simulink model "PMSM_temperature_estimation_EKF"  (R2023b)
settings: Solver=VariableStepAuto  StartTime=0.0  StopTime=10  FixedStep=dt  RelTol=1e-3  AbsTol=1e-3
values from neighbouring files (symbols this model uses):
  CF_fc = 1/(20*Ts)    (= 5)    [controller_parameters.m]
  CF_k = 1    [controller_parameters.m]
  dt = 50e-6    (= 5e-05)    [config.m]
  dt_speed_control = 0.001    [config.m]
  max_power = 50e3    (= 50000)    [config.m]
  max_torque = 220    [config.m]
  N = 6    [config.m]
  ratio_rotor = 0.75    [config.m]
  Rd_percent_rotor = ratio_rotor*100    (= 75)    [config.m]
  Rm_percent_rotor = ratio_rotor*100    (= 75)    [config.m]
  rotor_initial_temperatures = 298.15    [config.m]
  stator_initial_temperatures = [298.15;298.15;298.15]    [config.m]
  stator_thermal_mass = 100    [config.m]
  Ts = 0.01    [controller_parameters.m]
undefined symbols (not defined in the file or in its folder): cex, ch, cJ, DiscIntNeverNeededParam
libraries: fl_lib x152, nesl_utility x45, fl_ps_legacy_lib x3, sharedTrackingLibrary x1, ee_lib x1, SignalEditorBlockLib x1, simulink x1
(part 2 of 3)

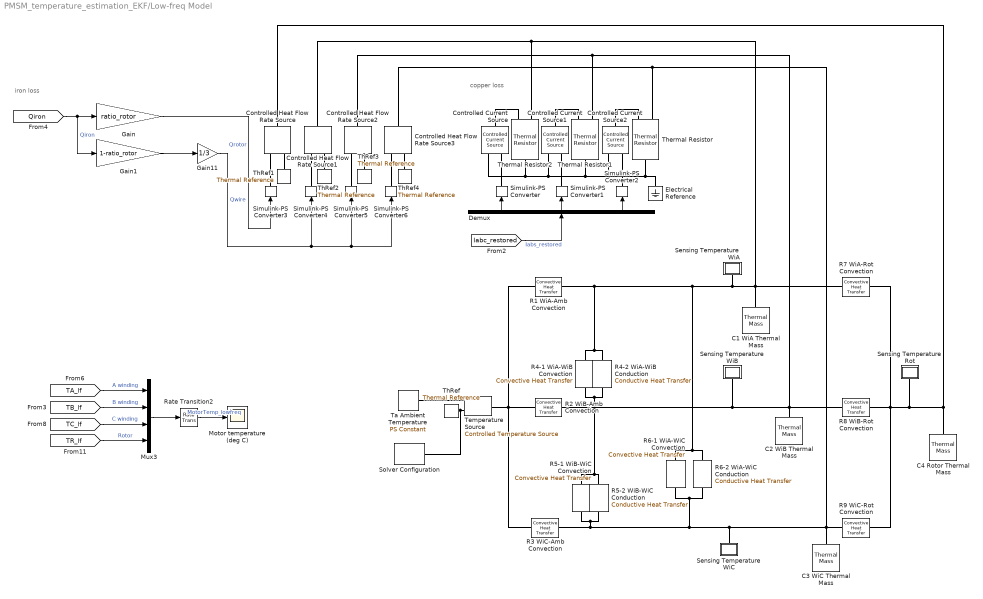
== system PMSM_temperature_estimation_EKF/Low-freq Model ==
  note: iron loss
  note: copper loss
  C1 WiA Thermal Mass : fl_lib/Thermal/Thermal Elements/Thermal Mass  mass_type=foundation.enum.constant_variable.constant  mass=1 kg  sp_heat=stator_thermal_mass J/(K*kg)  mass_min=1e-6 kg  num_ports=foundation.enum.numPorts2.one  m_specify=off  m_priority=High  m=1 kg  m_nominal_specify=off  m_nominal_unit=kg  m_nominal_value=1  T_specify=on  T_priority=High  T=stator_initial_temperatures(1) K  T_nominal_specify=off  T_nominal_unit=K  T_nominal_value=1  Q_specify=off  Q_priority=High  Q=0 W  Q_nominal_specify=off  Q_nominal_unit=W  Q_nominal_value=1
  C2 WiB Thermal Mass : fl_lib/Thermal/Thermal Elements/Thermal Mass  mass_type=foundation.enum.constant_variable.constant  mass=1 kg  sp_heat=stator_thermal_mass J/(K*kg)  mass_min=1e-6 kg  num_ports=foundation.enum.numPorts2.one  m_specify=off  m_priority=High  m=1 kg  m_nominal_specify=off  m_nominal_unit=kg  m_nominal_value=1  T_specify=on  T_priority=High  T=stator_initial_temperatures(2) K  T_nominal_specify=off  T_nominal_unit=K  T_nominal_value=1  Q_specify=off  Q_priority=High  Q=0 W  Q_nominal_specify=off  Q_nominal_unit=W  Q_nominal_value=1
  C3 WiC Thermal Mass : fl_lib/Thermal/Thermal Elements/Thermal Mass  mass_type=foundation.enum.constant_variable.constant  mass=1 kg  sp_heat=stator_thermal_mass J/(K*kg)  mass_min=1e-6 kg  num_ports=foundation.enum.numPorts2.one  m_specify=off  m_priority=High  m=1 kg  m_nominal_specify=off  m_nominal_unit=kg  m_nominal_value=1  T_specify=on  T_priority=High  T=stator_initial_temperatures(3) K  T_nominal_specify=off  T_nominal_unit=K  T_nominal_value=1  Q_specify=off  Q_priority=High  Q=0 W  Q_nominal_specify=off  Q_nominal_unit=W  Q_nominal_value=1
  C4 Rotor Thermal Mass : fl_lib/Thermal/Thermal Elements/Thermal Mass  mass_type=foundation.enum.constant_variable.constant  mass=1 kg  sp_heat=rotor_thermal_mass J/(K*kg)  mass_min=1e-6 kg  num_ports=foundation.enum.numPorts2.one  m_specify=off  m_priority=High  m=1 kg  m_nominal_specify=off  m_nominal_unit=kg  m_nominal_value=1  T_specify=on  T_priority=High  T=rotor_initial_temperatures K  T_nominal_specify=off  T_nominal_unit=K  T_nominal_value=1  Q_specify=off  Q_priority=High  Q=0 W  Q_nominal_specify=off  Q_nominal_unit=W  Q_nominal_value=1
  Controlled Current Source : fl_lib/Electrical/Electrical Sources/Controlled Current Source
  Controlled Current Source1 : fl_lib/Electrical/Electrical Sources/Controlled Current Source
  Controlled Current Source2 : fl_lib/Electrical/Electrical Sources/Controlled Current Source
  Controlled Heat Flow Rate Source{,1..3} (4 alike) : fl_lib/Thermal/Thermal Sources/Controlled Heat Flow Rate Source
  Demux : Demux  Outputs=3
  Electrical Reference : fl_lib/Electrical/Electrical Elements/Electrical Reference
  Gain : Gain  Gain=ratio_rotor
  Gain1 : Gain  Gain=1-ratio_rotor
  Gain11 : Gain  Gain=1/3
  Motor temperature (deg C) : Scope
  Mux3 : Mux
  R1 WiA-Amb Convection : fl_lib/Thermal/Thermal Elements/Convective Heat Transfer  thermal_type=foundation.enum.constant_variable.constant  area=0.1 m^2  heat_tr_coeff=20 W/(m^2 * K)  min_heat_tr_coeff=1e-3 W/(K*m^2)  T_specify=off  T_priority=None  T=0 K  T_nominal_specify=off  T_nominal_unit=K  T_nominal_value=1  Q_specify=off  Q_priority=None  Q=0 J/s  Q_nominal_specify=off  Q_nominal_unit=J/s  Q_nominal_value=1
  R2 WiB-Amb Convection : fl_lib/Thermal/Thermal Elements/Convective Heat Transfer  thermal_type=foundation.enum.constant_variable.constant  area=0.1 m^2  heat_tr_coeff=20 W/(m^2 * K)  min_heat_tr_coeff=1e-3 W/(K*m^2)  T_specify=off  T_priority=None  T=0 K  T_nominal_specify=off  T_nominal_unit=K  T_nominal_value=1  Q_specify=off  Q_priority=None  Q=0 J/s  Q_nominal_specify=off  Q_nominal_unit=J/s  Q_nominal_value=1
  R3 WiC-Amb Convection : fl_lib/Thermal/Thermal Elements/Convective Heat Transfer  thermal_type=foundation.enum.constant_variable.constant  area=0.1 m^2  heat_tr_coeff=20 W/(m^2 * K)  min_heat_tr_coeff=1e-3 W/(K*m^2)  T_specify=off  T_priority=None  T=0 K  T_nominal_specify=off  T_nominal_unit=K  T_nominal_value=1  Q_specify=off  Q_priority=None  Q=0 J/s  Q_nominal_specify=off  Q_nominal_unit=J/s  Q_nominal_value=1
  R4-1 WiA-WiB Convection : fl_lib/Thermal/Thermal Elements/Convective Heat Transfer  thermal_type=foundation.enum.constant_variable.constant  area=0.004 m^2  heat_tr_coeff=200 W/(m^2 * K)  min_heat_tr_coeff=1e-3 W/(K*m^2)  T_specify=off  T_priority=None  T=0 K  T_nominal_specify=off  T_nominal_unit=K  T_nominal_value=1  Q_specify=off  Q_priority=None  Q=0 J/s  Q_nominal_specify=off  Q_nominal_unit=J/s  Q_nominal_value=1
  R4-2 WiA-WiB Conduction : fl_lib/Thermal/Thermal Elements/Conductive Heat Transfer  thermal_type=foundation.enum.ConstantVariableTabulated.Constant  wall_geometry=foundation.enum.ConductionWallGeometry.Planar  area=0.002 m^2  thickness=0.1 m  d_in=0.05 m  d_out=0.1 m  L=1 m  th_cond_min=10 W/(K*m)  th_cond=80 W/(m*K)  th_cond_TLU=[413, 401, 392, 383, 371, 357, 342] W/(K*m)  temp_TLU=[200, 273, 400, 600, 800, 1000, 1200] K  T_specify=off  T_priority=None  T=0 K  T_nominal_specify=off  T_nominal_unit=K  T_nominal_value=1  Q_specify=off  Q_priority=None  Q=0 J/s  Q_nominal_specify=off  Q_nominal_unit=J/s  Q_nominal_value=1
  R5-1 WiB-WiC Convection : fl_lib/Thermal/Thermal Elements/Convective Heat Transfer  thermal_type=foundation.enum.constant_variable.constant  area=0.004 m^2  heat_tr_coeff=200 W/(m^2 * K)  min_heat_tr_coeff=1e-3 W/(K*m^2)  T_specify=off  T_priority=None  T=0 K  T_nominal_specify=off  T_nominal_unit=K  T_nominal_value=1  Q_specify=off  Q_priority=None  Q=0 J/s  Q_nominal_specify=off  Q_nominal_unit=J/s  Q_nominal_value=1
  R5-2 WiB-WiC Conduction : fl_lib/Thermal/Thermal Elements/Conductive Heat Transfer  thermal_type=foundation.enum.ConstantVariableTabulated.Constant  wall_geometry=foundation.enum.ConductionWallGeometry.Planar  area=0.002 m^2  thickness=0.1 m  d_in=0.05 m  d_out=0.1 m  L=1 m  th_cond_min=10 W/(K*m)  th_cond=80 W/(m*K)  th_cond_TLU=[413, 401, 392, 383, 371, 357, 342] W/(K*m)  temp_TLU=[200, 273, 400, 600, 800, 1000, 1200] K  T_specify=off  T_priority=None  T=0 K  T_nominal_specify=off  T_nominal_unit=K  T_nominal_value=1  Q_specify=off  Q_priority=None  Q=0 J/s  Q_nominal_specify=off  Q_nominal_unit=J/s  Q_nominal_value=1
  R6-1 WiA-WiC Convection : fl_lib/Thermal/Thermal Elements/Convective Heat Transfer  thermal_type=foundation.enum.constant_variable.constant  area=0.004 m^2  heat_tr_coeff=200 W/(m^2 * K)  min_heat_tr_coeff=1e-3 W/(K*m^2)  T_specify=off  T_priority=None  T=0 K  T_nominal_specify=off  T_nominal_unit=K  T_nominal_value=1  Q_specify=off  Q_priority=None  Q=0 J/s  Q_nominal_specify=off  Q_nominal_unit=J/s  Q_nominal_value=1
  R6-2 WiA-WiC Conduction : fl_lib/Thermal/Thermal Elements/Conductive Heat Transfer  thermal_type=foundation.enum.ConstantVariableTabulated.Constant  wall_geometry=foundation.enum.ConductionWallGeometry.Planar  area=0.002 m^2  thickness=0.1 m  d_in=0.05 m  d_out=0.1 m  L=1 m  th_cond_min=10 W/(K*m)  th_cond=80 W/(m*K)  th_cond_TLU=[413, 401, 392, 383, 371, 357, 342] W/(K*m)  temp_TLU=[200, 273, 400, 600, 800, 1000, 1200] K  T_specify=off  T_priority=None  T=0 K  T_nominal_specify=off  T_nominal_unit=K  T_nominal_value=1  Q_specify=off  Q_priority=None  Q=0 J/s  Q_nominal_specify=off  Q_nominal_unit=J/s  Q_nominal_value=1
  R7 WiA-Rot Convection : fl_lib/Thermal/Thermal Elements/Convective Heat Transfer  thermal_type=foundation.enum.constant_variable.constant  area=0.02 m^2  heat_tr_coeff=200 W/(m^2 * K)  min_heat_tr_coeff=1e-3 W/(K*m^2)  T_specify=off  T_priority=None  T=0 K  T_nominal_specify=off  T_nominal_unit=K  T_nominal_value=1  Q_specify=off  Q_priority=None  Q=0 J/s  Q_nominal_specify=off  Q_nominal_unit=J/s  Q_nominal_value=1
  R8 WiB-Rot Convection : fl_lib/Thermal/Thermal Elements/Convective Heat Transfer  thermal_type=foundation.enum.constant_variable.constant  area=0.02 m^2  heat_tr_coeff=200 W/(m^2 * K)  min_heat_tr_coeff=1e-3 W/(K*m^2)  T_specify=off  T_priority=None  T=0 K  T_nominal_specify=off  T_nominal_unit=K  T_nominal_value=1  Q_specify=off  Q_priority=None  Q=0 J/s  Q_nominal_specify=off  Q_nominal_unit=J/s  Q_nominal_value=1
  R9 WiC-Rot Convection : fl_lib/Thermal/Thermal Elements/Convective Heat Transfer  thermal_type=foundation.enum.constant_variable.constant  area=0.02 m^2  heat_tr_coeff=200 W/(m^2 * K)  min_heat_tr_coeff=1e-3 W/(K*m^2)  T_specify=off  T_priority=None  T=0 K  T_nominal_specify=off  T_nominal_unit=K  T_nominal_value=1  Q_specify=off  Q_priority=None  Q=0 J/s  Q_nominal_specify=off  Q_nominal_unit=J/s  Q_nominal_value=1
  Rate Transition2 : RateTransition  OutPortSampleTime=dt_display
  Sensing Temperature Rot : Subsystem
      mask Display: disp('TR')
  Sensing Temperature WiA : Subsystem
      mask Display: disp('TA')
  Sensing Temperature WiB : Subsystem
      mask Display: disp('TB')
  Sensing Temperature WiC : Subsystem
      mask Display: disp('TC')
  Simulink-PS Converter : nesl_utility/Simulink-PS Converter  PhysicalDomain=network_engine_domain  SubClassName=ps_input  LeftPortType=input  RightPortType=output  PseudoPeriodic=off  Frequencies=[]  NoiseDistribution=none  NoiseParameters=[]  Unit=A  AffineConversion=off  FilteringAndDerivatives=provide  SimscapeFilterOrder=1  InputFilterTimeConstant=0.001  UdotUserProvided=0
  Simulink-PS Converter1 : nesl_utility/Simulink-PS Converter  PhysicalDomain=network_engine_domain  SubClassName=ps_input  LeftPortType=input  RightPortType=output  PseudoPeriodic=off  Frequencies=[]  NoiseDistribution=none  NoiseParameters=[]  Unit=A  AffineConversion=off  FilteringAndDerivatives=provide  SimscapeFilterOrder=1  InputFilterTimeConstant=0.001  UdotUserProvided=0
  Simulink-PS Converter2 : nesl_utility/Simulink-PS Converter  PhysicalDomain=network_engine_domain  SubClassName=ps_input  LeftPortType=input  RightPortType=output  PseudoPeriodic=off  Frequencies=[]  NoiseDistribution=none  NoiseParameters=[]  Unit=A  AffineConversion=off  FilteringAndDerivatives=provide  SimscapeFilterOrder=1  InputFilterTimeConstant=0.001  UdotUserProvided=0
  Simulink-PS Converter{3..6} (4 alike) : nesl_utility/Simulink-PS Converter  PhysicalDomain=network_engine_domain  SubClassName=ps_input  LeftPortType=input  RightPortType=output  PseudoPeriodic=off  Frequencies=[]  NoiseDistribution=none  NoiseParameters=[]  Unit=J/s  AffineConversion=off  FilteringAndDerivatives=provide  SimscapeFilterOrder=1  InputFilterTimeConstant=0.001  UdotUserProvided=0
  Solver Configuration : nesl_utility/Solver Configuration  PhysicalDomain=network_engine_domain  SubClassName=solver  LeftPortType=input  RightPortType=generic  Tones=[]  Harmonics=[]  SimulateNoise=off  Profile=off  UseLocalSampling=off  EnableSwitchedLinearOptims=on  FrequencyDomain=off  UseCCode=off  RelTol=0.001  AbsTol=0.001  MinStep=1e-09  ToWorkspace=off  RevertToSquareIcSolve=off  NumHomotopyIterations=100  PhasorMode=off  PhasorModeNumHarmonics=1  ConsistencySolver=NEWTON_XTOL_AFTER_FTOL  IndexReductionMethod=DerivativeReplacement  DoDC=off  ResidualTolerance=1e-09  ConsistencyTolSource=GLOBAL  ConsistencyAbsTol=0.001  ConsistencyRelTol=0.001  ConsistencyTolFactor=0.001  UseLocalSolver=off  LocalSolverChoice=NE_BACKWARD_EULER_ADVANCER  ResolveIndetEquations=on  FunctionEvalNumThread=1  LocalSolverSampleTime=0.001  DoFixedCost=off  MaxNonlinIter=3  MaxModeIter=2  ComputeImpulses=off  ImpulseIterations=2  LinearAlgebra=auto  LinearAlgebraNumThread=0  EquationFormulation=NE_TIME_EF  DelaysMemoryBudget=1024  AutomaticFiltering=on  FilteringTimeConstant=0.001  PartitionStorageMethod=AS_NEEDED  PartitionMemoryBudget=1024  PartitionMethod=ROBUST  MultibodyUseLocalSolver=off  MultibodyLocalSolverChoice=ODE1  MultibodyLocalSolverSampleTime=0.001
  Ta Ambient Temperature : fl_lib/Physical Signals/Sources/PS Constant  constant=300
  Temperature Source : fl_lib/Thermal/Thermal Sources/Controlled Temperature Source
  ThRef{,1..4} (5 alike) : fl_lib/Thermal/Thermal Elements/Thermal Reference
  Thermal Resistor : fl_lib/Electrical/Electrical Elements/Thermal Resistor  R0=Rs Ohm  T0=Tmeas K  alpha=alpha 1/K  tc=0.1 s  K_d=1e-3 W/K  T_specify=on  T_priority=High  T=stator_initial_temperatures(3) K  T_nominal_specify=off  T_nominal_unit=K  T_nominal_value=1
      settings: InternalSimscapePortConfiguration="{\"Bottom\":[],\"Left\":[{\"id\":\"H\",\"label\":\"H\",\"type\":\"foundation.thermal.thermal\"},{\"id\":\"p\",\"label\":\"+\",\"type\":\"foundation.electrical.electrical\"}],\"Right\":[{\"id\":\"n\",\"label\":\"-\",\"type\":\"foundation.electrical.electrical\"}],\"Top\":[]}"
  Thermal Resistor1 : fl_lib/Electrical/Electrical Elements/Thermal Resistor  R0=Rs Ohm  T0=Tmeas K  alpha=alpha 1/K  tc=0.1 s  K_d=1e-3 W/K  T_specify=on  T_priority=High  T=stator_initial_temperatures(2) K  T_nominal_specify=off  T_nominal_unit=K  T_nominal_value=1
      settings: InternalSimscapePortConfiguration="{\"Bottom\":[],\"Left\":[{\"id\":\"H\",\"label\":\"H\",\"type\":\"foundation.thermal.thermal\"},{\"id\":\"p\",\"label\":\"+\",\"type\":\"foundation.electrical.electrical\"}],\"Right\":[{\"id\":\"n\",\"label\":\"-\",\"type\":\"foundation.electrical.electrical\"}],\"Top\":[]}"
  Thermal Resistor2 : fl_lib/Electrical/Electrical Elements/Thermal Resistor  R0=Rs Ohm  T0=Tmeas K  alpha=alpha 1/K  tc=0.1 s  K_d=1e-3 W/K  T_specify=on  T_priority=High  T=stator_initial_temperatures(1) K  T_nominal_specify=off  T_nominal_unit=K  T_nominal_value=1
      settings: InternalSimscapePortConfiguration="{\"Bottom\":[],\"Left\":[{\"id\":\"H\",\"label\":\"H\",\"type\":\"foundation.thermal.thermal\"},{\"id\":\"p\",\"label\":\"+\",\"type\":\"foundation.electrical.electrical\"}],\"Right\":[{\"id\":\"n\",\"label\":\"-\",\"type\":\"foundation.electrical.electrical\"}],\"Top\":[]}"
  wires:
  Rate Transition2/1 -> Motor temperature (deg C)/1  "MotorTemp_lowfreq"
  [TA_lf] -> Mux3/1  "A winding"
  [TR_lf] -> Mux3/4  "Rotor"
  [TC_lf] -> Mux3/3  "C winding"
  [TB_lf] -> Mux3/2  "B winding"
  Mux3/1 -> Rate Transition2/1
  Gain11/1 -> Simulink-PS Converter4/1, Simulink-PS Converter6/1, Simulink-PS Converter5/1  "Qwire"
  Gain/1 -> Simulink-PS Converter3/1  "Qrotor"
  Demux/1 -> Simulink-PS Converter/1
  Demux/2 -> Simulink-PS Converter1/1
  Demux/3 -> Simulink-PS Converter2/1
  [Iabc_restored] -> Demux/1  "Iabs_restored"
  [Qiron] -> Gain1/1, Gain/1  "Qiron"
  Gain1/1 -> Gain11/1
  connections:
  R7 WiA-Rot Convection/RConn1 -- Sensing Temperature WiA/LConn1 -- R6-1 WiA-WiC Convection/RConn1 -- R6-2 WiA-WiC Conduction/RConn1 -- R4-1 WiA-WiB Convection/LConn1 -- R4-2 WiA-WiB Conduction/LConn1 -- R1 WiA-Amb Convection/LConn1 -- Controlled Heat Flow Rate Source1/LConn1 -- Thermal Resistor2/LConn1 -- C1 WiA Thermal Mass/LConn1
  Sensing Temperature Rot/LConn1 -- Controlled Heat Flow Rate Source/LConn1 -- C4 Rotor Thermal Mass/LConn1 -- R8 WiB-Rot Convection/LConn1 -- R7 WiA-Rot Convection/LConn1 -- R9 WiC-Rot Convection/LConn1
  R4-1 WiA-WiB Convection/RConn1 -- R4-2 WiA-WiB Conduction/RConn1 -- R8 WiB-Rot Convection/RConn1 -- Controlled Heat Flow Rate Source2/LConn1 -- Thermal Resistor1/LConn1 -- C2 WiB Thermal Mass/LConn1 -- Sensing Temperature WiB/LConn1 -- R2 WiB-Amb Convection/LConn1 -- R5-1 WiB-WiC Convection/LConn1 -- R5-2 WiB-WiC Conduction/LConn1
  R9 WiC-Rot Convection/RConn1 -- R5-2 WiB-WiC Conduction/RConn1 -- R5-1 WiB-WiC Convection/RConn1 -- R3 WiC-Amb Convection/LConn1 -- R6-1 WiA-WiC Convection/LConn1 -- R6-2 WiA-WiC Conduction/LConn1 -- Sensing Temperature WiC/LConn1 -- Controlled Heat Flow Rate Source3/LConn1 -- Thermal Resistor/LConn1 -- C3 WiC Thermal Mass/LConn1
  R1 WiA-Amb Convection/RConn1 -- Temperature Source/LConn1 -- R3 WiC-Amb Convection/RConn1 -- R2 WiB-Amb Convection/RConn1
  Ta Ambient Temperature/RConn1 -- Temperature Source/RConn1
  ThRef/LConn1 -- Solver Configuration/RConn1 -- Temperature Source/RConn2
  Thermal Resistor/RConn1 -- Electrical Reference/LConn1 -- Controlled Current Source2/RConn2 -- Controlled Current Source/RConn2 -- Thermal Resistor2/RConn1 -- Controlled Current Source1/RConn2 -- Thermal Resistor1/RConn1
  Controlled Current Source/LConn1 -- Thermal Resistor2/LConn2
  Controlled Current Source1/LConn1 -- Thermal Resistor1/LConn2
  Controlled Current Source2/LConn1 -- Thermal Resistor/LConn2
  Simulink-PS Converter/RConn1 -- Controlled Current Source/RConn1
  Simulink-PS Converter1/RConn1 -- Controlled Current Source1/RConn1
  Controlled Current Source2/RConn1 -- Simulink-PS Converter2/RConn1
  ThRef1/LConn1 -- Controlled Heat Flow Rate Source/RConn2
  Simulink-PS Converter3/RConn1 -- Controlled Heat Flow Rate Source/RConn1
  Simulink-PS Converter4/RConn1 -- Controlled Heat Flow Rate Source1/RConn1
  ThRef2/LConn1 -- Controlled Heat Flow Rate Source1/RConn2
  ThRef3/LConn1 -- Controlled Heat Flow Rate Source2/RConn2
  Controlled Heat Flow Rate Source2/RConn1 -- Simulink-PS Converter5/RConn1
  Controlled Heat Flow Rate Source3/RConn1 -- Simulink-PS Converter6/RConn1
  ThRef4/LConn1 -- Controlled Heat Flow Rate Source3/RConn2

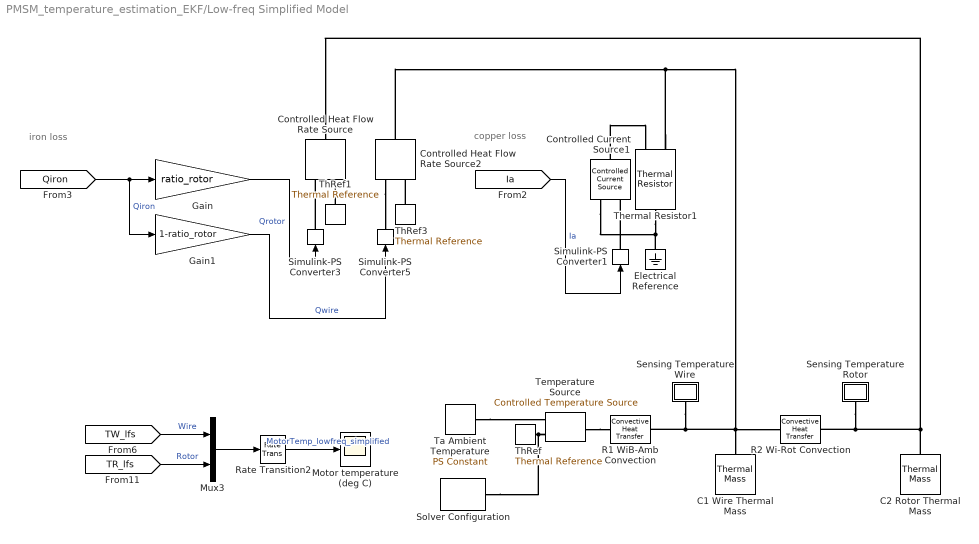
== system PMSM_temperature_estimation_EKF/Low-freq Simplified Model ==
  note: iron loss
  note: copper loss
  C1 Wire Thermal Mass : fl_lib/Thermal/Thermal Elements/Thermal Mass  mass_type=foundation.enum.constant_variable.constant  mass=1 kg  sp_heat=3*stator_thermal_mass J/(K*kg)  mass_min=1e-6 kg  num_ports=foundation.enum.numPorts2.one  m_specify=off  m_priority=High  m=1 kg  m_nominal_specify=off  m_nominal_unit=kg  m_nominal_value=1  T_specify=on  T_priority=High  T=mean(stator_initial_temperatures) K  T_nominal_specify=off  T_nominal_unit=K  T_nominal_value=1  Q_specify=off  Q_priority=High  Q=0 W  Q_nominal_specify=off  Q_nominal_unit=W  Q_nominal_value=1
  C2 Rotor Thermal Mass : fl_lib/Thermal/Thermal Elements/Thermal Mass  mass_type=foundation.enum.constant_variable.constant  mass=1 kg  sp_heat=rotor_thermal_mass J/(K*kg)  mass_min=1e-6 kg  num_ports=foundation.enum.numPorts2.one  m_specify=off  m_priority=High  m=1 kg  m_nominal_specify=off  m_nominal_unit=kg  m_nominal_value=1  T_specify=on  T_priority=High  T=rotor_initial_temperatures K  T_nominal_specify=off  T_nominal_unit=K  T_nominal_value=1  Q_specify=off  Q_priority=High  Q=0 W  Q_nominal_specify=off  Q_nominal_unit=W  Q_nominal_value=1
  Controlled Current Source1 : fl_lib/Electrical/Electrical Sources/Controlled Current Source
  Controlled Heat Flow Rate Source : fl_lib/Thermal/Thermal Sources/Controlled Heat Flow Rate Source
  Controlled Heat Flow Rate Source2 : fl_lib/Thermal/Thermal Sources/Controlled Heat Flow Rate Source
  Electrical Reference : fl_lib/Electrical/Electrical Elements/Electrical Reference
  Gain : Gain  Gain=ratio_rotor
  Gain1 : Gain  Gain=1-ratio_rotor
  Motor temperature (deg C) : Scope
  Mux3 : Mux  Inputs=2
  R1 WiB-Amb Convection : fl_lib/Thermal/Thermal Elements/Convective Heat Transfer  thermal_type=foundation.enum.constant_variable.constant  area=3*0.1 m^2  heat_tr_coeff=20 W/(m^2 * K)  min_heat_tr_coeff=1e-3 W/(K*m^2)  T_specify=off  T_priority=None  T=0 K  T_nominal_specify=off  T_nominal_unit=K  T_nominal_value=1  Q_specify=off  Q_priority=None  Q=0 J/s  Q_nominal_specify=off  Q_nominal_unit=J/s  Q_nominal_value=1
  R2 Wi-Rot Convection : fl_lib/Thermal/Thermal Elements/Convective Heat Transfer  thermal_type=foundation.enum.constant_variable.constant  area=3*0.02 m^2  heat_tr_coeff=200 W/(m^2 * K)  min_heat_tr_coeff=1e-3 W/(K*m^2)  T_specify=off  T_priority=None  T=0 K  T_nominal_specify=off  T_nominal_unit=K  T_nominal_value=1  Q_specify=off  Q_priority=None  Q=0 J/s  Q_nominal_specify=off  Q_nominal_unit=J/s  Q_nominal_value=1
  Rate Transition2 : RateTransition  OutPortSampleTime=dt_display
  Sensing Temperature Rotor : Subsystem
      mask Display: disp('TR')
  Sensing Temperature Wire : Subsystem
      mask Display: disp('TW')
  Simulink-PS Converter1 : nesl_utility/Simulink-PS Converter  PhysicalDomain=network_engine_domain  SubClassName=ps_input  LeftPortType=input  RightPortType=output  PseudoPeriodic=off  Frequencies=[]  NoiseDistribution=none  NoiseParameters=[]  Unit=A  AffineConversion=off  FilteringAndDerivatives=provide  SimscapeFilterOrder=1  InputFilterTimeConstant=0.001  UdotUserProvided=0
  Simulink-PS Converter3 : nesl_utility/Simulink-PS Converter  PhysicalDomain=network_engine_domain  SubClassName=ps_input  LeftPortType=input  RightPortType=output  PseudoPeriodic=off  Frequencies=[]  NoiseDistribution=none  NoiseParameters=[]  Unit=J/s  AffineConversion=off  FilteringAndDerivatives=provide  SimscapeFilterOrder=1  InputFilterTimeConstant=0.001  UdotUserProvided=0
  Simulink-PS Converter5 : nesl_utility/Simulink-PS Converter  PhysicalDomain=network_engine_domain  SubClassName=ps_input  LeftPortType=input  RightPortType=output  PseudoPeriodic=off  Frequencies=[]  NoiseDistribution=none  NoiseParameters=[]  Unit=J/s  AffineConversion=off  FilteringAndDerivatives=provide  SimscapeFilterOrder=1  InputFilterTimeConstant=0.001  UdotUserProvided=0
  Solver Configuration : nesl_utility/Solver Configuration  PhysicalDomain=network_engine_domain  SubClassName=solver  LeftPortType=input  RightPortType=generic  Tones=[]  Harmonics=[]  SimulateNoise=off  Profile=off  UseLocalSampling=off  EnableSwitchedLinearOptims=on  FrequencyDomain=off  UseCCode=off  RelTol=0.001  AbsTol=0.001  MinStep=1e-09  ToWorkspace=off  RevertToSquareIcSolve=off  NumHomotopyIterations=100  PhasorMode=off  PhasorModeNumHarmonics=1  ConsistencySolver=NEWTON_XTOL_AFTER_FTOL  IndexReductionMethod=DerivativeReplacement  DoDC=off  ResidualTolerance=1e-09  ConsistencyTolSource=GLOBAL  ConsistencyAbsTol=0.001  ConsistencyRelTol=0.001  ConsistencyTolFactor=0.001  UseLocalSolver=off  LocalSolverChoice=NE_BACKWARD_EULER_ADVANCER  ResolveIndetEquations=on  FunctionEvalNumThread=1  LocalSolverSampleTime=0.001  DoFixedCost=off  MaxNonlinIter=3  MaxModeIter=2  ComputeImpulses=off  ImpulseIterations=2  LinearAlgebra=auto  LinearAlgebraNumThread=0  EquationFormulation=NE_TIME_EF  DelaysMemoryBudget=1024  AutomaticFiltering=on  FilteringTimeConstant=0.001  PartitionStorageMethod=AS_NEEDED  PartitionMemoryBudget=1024  PartitionMethod=ROBUST  MultibodyUseLocalSolver=off  MultibodyLocalSolverChoice=ODE1  MultibodyLocalSolverSampleTime=0.001
  Ta Ambient Temperature : fl_lib/Physical Signals/Sources/PS Constant  constant=300
  Temperature Source : fl_lib/Thermal/Thermal Sources/Controlled Temperature Source
  ThRef : fl_lib/Thermal/Thermal Elements/Thermal Reference
  ThRef1 : fl_lib/Thermal/Thermal Elements/Thermal Reference
  ThRef3 : fl_lib/Thermal/Thermal Elements/Thermal Reference
  Thermal Resistor1 : fl_lib/Electrical/Electrical Elements/Thermal Resistor  R0=Rs Ohm  T0=Tmeas K  alpha=alpha 1/K  tc=0.1 s  K_d=1e-3 W/K  T_specify=on  T_priority=High  T=stator_initial_temperatures(2) K  T_nominal_specify=off  T_nominal_unit=K  T_nominal_value=1
      settings: InternalSimscapePortConfiguration="{\"Bottom\":[],\"Left\":[{\"id\":\"H\",\"label\":\"H\",\"type\":\"foundation.thermal.thermal\"},{\"id\":\"p\",\"label\":\"+\",\"type\":\"foundation.electrical.electrical\"}],\"Right\":[{\"id\":\"n\",\"label\":\"-\",\"type\":\"foundation.electrical.electrical\"}],\"Top\":[]}"
  wires:
  Rate Transition2/1 -> Motor temperature (deg C)/1  "MotorTemp_lowfreq_simplified"
  [TW_lfs] -> Mux3/1  "Wire"
  [TR_lfs] -> Mux3/2  "Rotor"
  Mux3/1 -> Rate Transition2/1
  Gain1/1 -> Simulink-PS Converter5/1  "Qwire"
  Gain/1 -> Simulink-PS Converter3/1  "Qrotor"
  [Ia] -> Simulink-PS Converter1/1  "Ia"
  [Qiron] -> Gain1/1, Gain/1  "Qiron"
  connections:
  R2 Wi-Rot Convection/LConn1 -- C2 Rotor Thermal Mass/LConn1 -- Controlled Heat Flow Rate Source/LConn1 -- Sensing Temperature Rotor/LConn1
  Controlled Heat Flow Rate Source2/LConn1 -- Sensing Temperature Wire/LConn1 -- R1 WiB-Amb Convection/LConn1 -- C1 Wire Thermal Mass/LConn1 -- R2 Wi-Rot Convection/RConn1 -- Thermal Resistor1/LConn1
  Temperature Source/LConn1 -- R1 WiB-Amb Convection/RConn1
  Ta Ambient Temperature/RConn1 -- Temperature Source/RConn1
  Temperature Source/RConn2 -- ThRef/LConn1 -- Solver Configuration/RConn1
  Controlled Current Source1/RConn2 -- Electrical Reference/LConn1 -- Thermal Resistor1/RConn1
  Controlled Current Source1/LConn1 -- Thermal Resistor1/LConn2
  Simulink-PS Converter1/RConn1 -- Controlled Current Source1/RConn1
  ThRef1/LConn1 -- Controlled Heat Flow Rate Source/RConn2
  Simulink-PS Converter3/RConn1 -- Controlled Heat Flow Rate Source/RConn1
  ThRef3/LConn1 -- Controlled Heat Flow Rate Source2/RConn2
  Controlled Heat Flow Rate Source2/RConn1 -- Simulink-PS Converter5/RConn1

== system PMSM_temperature_estimation_EKF/PMSM Controller ==
  imeas : Inport
  theta : Inport  Port=2
  trqRef : Inport  Port=3
  Rate Transition : RateTransition
  Vector controller : Subsystem  mask(Vector controller){Np=6, lambda=0.1, h=10}
      mask prompts: Np "Number of pole pairs, p"; lambda "Flux linkage from rotor permanent magnet"; h "Current hysteresis (A)"
  G : Outport  VectorParamsAs1DForOutWhenUnconnected=off
  tag scope: trqDemand=global
  wires:
  theta/1 -> Vector controller/2(theta)
  imeas/1 -> Vector controller/3(I_abc)
  trqRef/1 -> Rate Transition/1
  Vector controller/1(G) -> G/1
  Rate Transition/1 -> Vector controller/1(trqRef), [trqDemand]

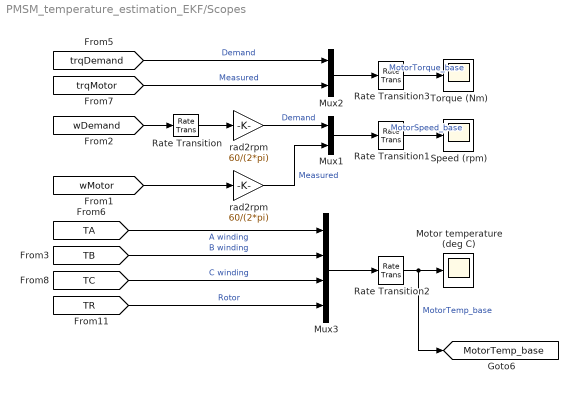
== system PMSM_temperature_estimation_EKF/Scopes ==
  " rad2rpm " : Gain  Gain=60/(2*pi)
  Motor temperature (deg C) : Scope
  Mux1 : Mux  Inputs=2
  Mux2 : Mux  Inputs=2
  Mux3 : Mux
  Rate Transition : RateTransition
  Rate Transition1 : RateTransition  OutPortSampleTime=dt_display
  Rate Transition2 : RateTransition  OutPortSampleTime=dt_display
  Rate Transition3 : RateTransition  OutPortSampleTime=dt_display
  Speed (rpm) : Scope
  Torque (Nm) : Scope
  rad2rpm : Gain  Gain=60/(2*pi)
  tag scope: MotorTemp_base=global
  wires:
  [trqDemand] -> Mux2/1  "Demand"
  [trqMotor] -> Mux2/2  "Measured"
  Mux2/1 -> Rate Transition3/1
  rad2rpm/1 -> Mux1/1  "Demand"
  " rad2rpm "/1 -> Mux1/2  "Measured"
  Mux1/1 -> Rate Transition1/1
  [wMotor] -> " rad2rpm "/1
  [wDemand] -> Rate Transition/1
  [TA] -> Mux3/1  "A winding"
  [TB] -> Mux3/2  "B winding"
  [TC] -> Mux3/3  "C winding"
  [TR] -> Mux3/4  "Rotor"
  Rate Transition2/1 -> [MotorTemp_base], Motor temperature (deg C)/1  "MotorTemp_base"
  Rate Transition/1 -> rad2rpm/1
  Rate Transition3/1 -> Torque (Nm)/1  "MotorTorque_base"
  Rate Transition1/1 -> Speed (rpm)/1  "MotorSpeed_base"
  Mux3/1 -> Rate Transition2/1

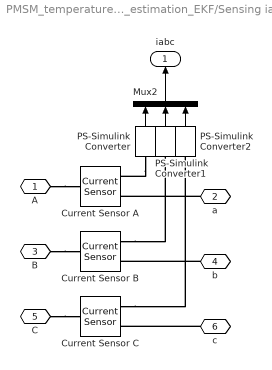
== system PMSM_temperature_estimation_EKF/Sensing iabc ==
  Current Sensor A : fl_lib/Electrical/Electrical Sensors/Current Sensor
  Current Sensor B : fl_lib/Electrical/Electrical Sensors/Current Sensor
  Current Sensor C : fl_lib/Electrical/Electrical Sensors/Current Sensor
  Mux2 : Mux  Inputs=[1,1,1]
  PS-Simulink Converter : nesl_utility/PS-Simulink Converter  PhysicalDomain=network_engine_domain  SubClassName=ps_output  LeftPortType=input  RightPortType=output  PseudoPeriodic=off  Frequencies=[]  VectorFormat=1-D array  Unit=A  AffineConversion=off
  PS-Simulink Converter1 : nesl_utility/PS-Simulink Converter  PhysicalDomain=network_engine_domain  SubClassName=ps_output  LeftPortType=input  RightPortType=output  PseudoPeriodic=off  Frequencies=[]  VectorFormat=1-D array  Unit=A  AffineConversion=off
  PS-Simulink Converter2 : nesl_utility/PS-Simulink Converter  PhysicalDomain=network_engine_domain  SubClassName=ps_output  LeftPortType=input  RightPortType=output  PseudoPeriodic=off  Frequencies=[]  VectorFormat=1-D array  Unit=A  AffineConversion=off
  A : PMIOPort  Side=Left
  a : PMIOPort  Port=2  Side=Right
  B : PMIOPort  Port=3  Side=Left
  b : PMIOPort  Port=4  Side=Right
  C : PMIOPort  Port=5  Side=Left
  c : PMIOPort  Port=6  Side=Right
  iabc : Outport  VectorParamsAs1DForOutWhenUnconnected=off
  wires:
  PS-Simulink Converter/1 -> Mux2/1
  PS-Simulink Converter1/1 -> Mux2/2
  PS-Simulink Converter2/1 -> Mux2/3
  Mux2/1 -> iabc/1
  connections:
  b/RConn1 -- Current Sensor B/RConn2
  A/RConn1 -- Current Sensor A/LConn1
  c/RConn1 -- Current Sensor C/RConn2
  Current Sensor B/RConn1 -- PS-Simulink Converter1/LConn1
  Current Sensor C/RConn1 -- PS-Simulink Converter2/LConn1
  a/RConn1 -- Current Sensor A/RConn2
  C/RConn1 -- Current Sensor C/LConn1
  PS-Simulink Converter/LConn1 -- Current Sensor A/RConn1
  B/RConn1 -- Current Sensor B/LConn1

== system PMSM_temperature_estimation_EKF/Speed Controller ==
  wMeas : Inport
  wRef : Inport  Port=2
  Power and torque limits : Subsystem
  Speed controller : Subsystem
  trqRef : Outport  VectorParamsAs1DForOutWhenUnconnected=off
  wires:
  Speed controller/1(trqRef) -> Power and torque limits/2(trqRef)
  wRef/1 -> Speed controller/2(wRef)
  wMeas/1 -> Power and torque limits/1(wMeas), Speed controller/1(wMeas)
  Power and torque limits/1(trqRefLim) -> trqRef/1

== system PMSM_temperature_estimation_EKF/State Space Model ==
  Bias : Bias  Bias=-273.15  SaturateOnIntegerOverflow=off
  Integrator : Integrator  InitialCondition=[stator_initial_temperatures;rotor_initial_temperatures]
  MATLAB Function : MATLAB Function  TreatAsAtomicUnit=on
  Mux : Mux  Inputs=3
  Rate Transition6 : RateTransition  OutPortSampleTime=dt_display
  Ta : Constant  Value=300  SampleTime=Ts
  Terminator1 : Terminator
  wires:
  [Iabc_restored] -> Mux/1  "Iabc"
  Ta/1 -> Mux/2  "Ta"
  [Qiron] -> Mux/3  "Qiron"
  MATLAB Function/1(dxdt) -> Integrator/1
  Integrator/1 -> Bias/1, MATLAB Function/1(x)
  Bias/1 -> Rate Transition6/1
  Rate Transition6/1 -> Terminator1/1  "MotorTemp_ss"
  Mux/1 -> MATLAB Function/2(u)  "u"

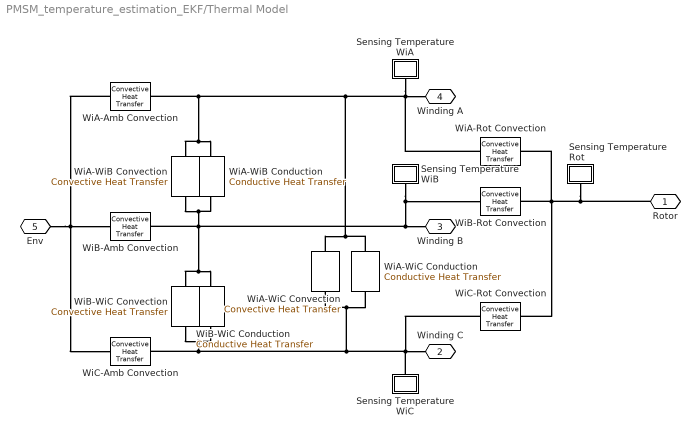
== system PMSM_temperature_estimation_EKF/Thermal Model ==
  Sensing Temperature Rot : Subsystem
      mask Display: disp('TR')
  Sensing Temperature WiA : Subsystem
      mask Display: disp('TA')
  Sensing Temperature WiB : Subsystem
      mask Display: disp('TB')
  Sensing Temperature WiC : Subsystem
      mask Display: disp('TC')
  WiA-Amb Convection : fl_lib/Thermal/Thermal Elements/Convective Heat Transfer  thermal_type=foundation.enum.constant_variable.constant  area=0.1 m^2  heat_tr_coeff=20 W/(m^2 * K)  min_heat_tr_coeff=1e-3 W/(K*m^2)  T_specify=off  T_priority=None  T=0 K  T_nominal_specify=off  T_nominal_unit=K  T_nominal_value=1  Q_specify=off  Q_priority=None  Q=0 J/s  Q_nominal_specify=off  Q_nominal_unit=J/s  Q_nominal_value=1
  WiA-Rot Convection : fl_lib/Thermal/Thermal Elements/Convective Heat Transfer  thermal_type=foundation.enum.constant_variable.constant  area=0.02 m^2  heat_tr_coeff=200 W/(m^2 * K)  min_heat_tr_coeff=1e-3 W/(K*m^2)  T_specify=off  T_priority=None  T=0 K  T_nominal_specify=off  T_nominal_unit=K  T_nominal_value=1  Q_specify=off  Q_priority=None  Q=0 J/s  Q_nominal_specify=off  Q_nominal_unit=J/s  Q_nominal_value=1
  WiA-WiB Conduction : fl_lib/Thermal/Thermal Elements/Conductive Heat Transfer  thermal_type=foundation.enum.ConstantVariableTabulated.Constant  wall_geometry=foundation.enum.ConductionWallGeometry.Planar  area=0.002 m^2  thickness=0.1 m  d_in=0.05 m  d_out=0.1 m  L=1 m  th_cond_min=10 W/(K*m)  th_cond=80 W/(m*K)  th_cond_TLU=[413, 401, 392, 383, 371, 357, 342] W/(K*m)  temp_TLU=[200, 273, 400, 600, 800, 1000, 1200] K  T_specify=off  T_priority=None  T=0 K  T_nominal_specify=off  T_nominal_unit=K  T_nominal_value=1  Q_specify=off  Q_priority=None  Q=0 J/s  Q_nominal_specify=off  Q_nominal_unit=J/s  Q_nominal_value=1
  WiA-WiB Convection : fl_lib/Thermal/Thermal Elements/Convective Heat Transfer  thermal_type=foundation.enum.constant_variable.constant  area=0.004 m^2  heat_tr_coeff=200 W/(m^2 * K)  min_heat_tr_coeff=1e-3 W/(K*m^2)  T_specify=off  T_priority=None  T=0 K  T_nominal_specify=off  T_nominal_unit=K  T_nominal_value=1  Q_specify=off  Q_priority=None  Q=0 J/s  Q_nominal_specify=off  Q_nominal_unit=J/s  Q_nominal_value=1
  WiA-WiC Conduction : fl_lib/Thermal/Thermal Elements/Conductive Heat Transfer  thermal_type=foundation.enum.ConstantVariableTabulated.Constant  wall_geometry=foundation.enum.ConductionWallGeometry.Planar  area=0.002 m^2  thickness=0.1 m  d_in=0.05 m  d_out=0.1 m  L=1 m  th_cond_min=10 W/(K*m)  th_cond=80 W/(m*K)  th_cond_TLU=[413, 401, 392, 383, 371, 357, 342] W/(K*m)  temp_TLU=[200, 273, 400, 600, 800, 1000, 1200] K  T_specify=off  T_priority=None  T=0 K  T_nominal_specify=off  T_nominal_unit=K  T_nominal_value=1  Q_specify=off  Q_priority=None  Q=0 J/s  Q_nominal_specify=off  Q_nominal_unit=J/s  Q_nominal_value=1
  WiA-WiC Convection : fl_lib/Thermal/Thermal Elements/Convective Heat Transfer  thermal_type=foundation.enum.constant_variable.constant  area=0.004 m^2  heat_tr_coeff=200 W/(m^2 * K)  min_heat_tr_coeff=1e-3 W/(K*m^2)  T_specify=off  T_priority=None  T=0 K  T_nominal_specify=off  T_nominal_unit=K  T_nominal_value=1  Q_specify=off  Q_priority=None  Q=0 J/s  Q_nominal_specify=off  Q_nominal_unit=J/s  Q_nominal_value=1
  WiB-Amb Convection : fl_lib/Thermal/Thermal Elements/Convective Heat Transfer  thermal_type=foundation.enum.constant_variable.constant  area=0.1 m^2  heat_tr_coeff=20 W/(m^2 * K)  min_heat_tr_coeff=1e-3 W/(K*m^2)  T_specify=off  T_priority=None  T=0 K  T_nominal_specify=off  T_nominal_unit=K  T_nominal_value=1  Q_specify=off  Q_priority=None  Q=0 J/s  Q_nominal_specify=off  Q_nominal_unit=J/s  Q_nominal_value=1
  WiB-Rot Convection : fl_lib/Thermal/Thermal Elements/Convective Heat Transfer  thermal_type=foundation.enum.constant_variable.constant  area=0.02 m^2  heat_tr_coeff=200 W/(m^2 * K)  min_heat_tr_coeff=1e-3 W/(K*m^2)  T_specify=off  T_priority=None  T=0 K  T_nominal_specify=off  T_nominal_unit=K  T_nominal_value=1  Q_specify=off  Q_priority=None  Q=0 J/s  Q_nominal_specify=off  Q_nominal_unit=J/s  Q_nominal_value=1
  WiB-WiC Conduction : fl_lib/Thermal/Thermal Elements/Conductive Heat Transfer  thermal_type=foundation.enum.ConstantVariableTabulated.Constant  wall_geometry=foundation.enum.ConductionWallGeometry.Planar  area=0.002 m^2  thickness=0.1 m  d_in=0.05 m  d_out=0.1 m  L=1 m  th_cond_min=10 W/(K*m)  th_cond=80 W/(m*K)  th_cond_TLU=[413, 401, 392, 383, 371, 357, 342] W/(K*m)  temp_TLU=[200, 273, 400, 600, 800, 1000, 1200] K  T_specify=off  T_priority=None  T=0 K  T_nominal_specify=off  T_nominal_unit=K  T_nominal_value=1  Q_specify=off  Q_priority=None  Q=0 J/s  Q_nominal_specify=off  Q_nominal_unit=J/s  Q_nominal_value=1
  WiB-WiC Convection : fl_lib/Thermal/Thermal Elements/Convective Heat Transfer  thermal_type=foundation.enum.constant_variable.constant  area=0.004 m^2  heat_tr_coeff=200 W/(m^2 * K)  min_heat_tr_coeff=1e-3 W/(K*m^2)  T_specify=off  T_priority=None  T=0 K  T_nominal_specify=off  T_nominal_unit=K  T_nominal_value=1  Q_specify=off  Q_priority=None  Q=0 J/s  Q_nominal_specify=off  Q_nominal_unit=J/s  Q_nominal_value=1
  WiC-Amb Convection : fl_lib/Thermal/Thermal Elements/Convective Heat Transfer  thermal_type=foundation.enum.constant_variable.constant  area=0.1 m^2  heat_tr_coeff=20 W/(m^2 * K)  min_heat_tr_coeff=1e-3 W/(K*m^2)  T_specify=off  T_priority=None  T=0 K  T_nominal_specify=off  T_nominal_unit=K  T_nominal_value=1  Q_specify=off  Q_priority=None  Q=0 J/s  Q_nominal_specify=off  Q_nominal_unit=J/s  Q_nominal_value=1
  WiC-Rot Convection : fl_lib/Thermal/Thermal Elements/Convective Heat Transfer  thermal_type=foundation.enum.constant_variable.constant  area=0.02 m^2  heat_tr_coeff=200 W/(m^2 * K)  min_heat_tr_coeff=1e-3 W/(K*m^2)  T_specify=off  T_priority=None  T=0 K  T_nominal_specify=off  T_nominal_unit=K  T_nominal_value=1  Q_specify=off  Q_priority=None  Q=0 J/s  Q_nominal_specify=off  Q_nominal_unit=J/s  Q_nominal_value=1
  Rotor : PMIOPort  Side=Left
  Winding C : PMIOPort  Port=2  Side=Right
  Winding B : PMIOPort  Port=3  Side=Right
  Winding A : PMIOPort  Port=4  Side=Right
  Env : PMIOPort  Port=5  Side=Left
  connections:
  WiA-Rot Convection/RConn1 -- WiA-WiC Conduction/RConn1 -- WiA-WiC Convection/RConn1 -- WiA-WiB Convection/LConn1 -- WiA-WiB Conduction/LConn1 -- WiA-Amb Convection/LConn1 -- Sensing Temperature WiA/LConn1 -- Winding A/RConn1
  Rotor/RConn1 -- Sensing Temperature Rot/LConn1 -- WiC-Rot Convection/LConn1 -- WiB-Rot Convection/LConn1 -- WiA-Rot Convection/LConn1
  WiA-WiB Convection/RConn1 -- WiA-WiB Conduction/RConn1 -- Sensing Temperature WiB/LConn1 -- WiB-Rot Convection/RConn1 -- Winding B/RConn1 -- WiB-Amb Convection/LConn1 -- WiB-WiC Conduction/LConn1 -- WiB-WiC Convection/LConn1
  WiC-Rot Convection/RConn1 -- Winding C/RConn1 -- WiB-WiC Conduction/RConn1 -- WiB-WiC Convection/RConn1 -- WiC-Amb Convection/LConn1 -- WiA-WiC Convection/LConn1 -- WiA-WiC Conduction/LConn1 -- Sensing Temperature WiC/LConn1
  WiA-Amb Convection/RConn1 -- Env/RConn1 -- WiC-Amb Convection/RConn1 -- WiB-Amb Convection/RConn1

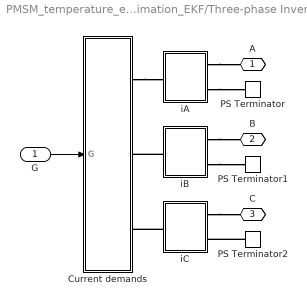
== system PMSM_temperature_estimation_EKF/Three-phase Inverter ==
  G : Inport
  Current demands : Subsystem
  PS Terminator : fl_lib/Physical Signals/Sinks/PS Terminator
  PS Terminator1 : fl_lib/Physical Signals/Sinks/PS Terminator
  PS Terminator2 : fl_lib/Physical Signals/Sinks/PS Terminator
  iA : Subsystem
  iB : Subsystem
  iC : Subsystem
  A : PMIOPort  Tag=PMCPort  Side=Right
  B : PMIOPort  Tag=PMCPort  Port=2  Side=Right
  C : PMIOPort  Tag=PMCPort  Port=3  Side=Right
  wires:
  G/1 -> Current demands/1(G)
  connections:
  iA/RConn1 -- A/RConn1
  Current demands/RConn1 -- iA/LConn1
  iB/LConn1 -- Current demands/RConn2
  iC/LConn1 -- Current demands/RConn3
  iB/RConn1 -- B/RConn1
  iC/RConn1 -- C/RConn1
  iA/RConn2 -- PS Terminator/LConn1
  PS Terminator2/LConn1 -- iC/RConn2
  iB/RConn2 -- PS Terminator1/LConn1

== system PMSM_temperature_estimation_EKF/Equivalent Model/Sensing Temperature Rot ==
  PS-Simulink Converter : nesl_utility/PS-Simulink Converter  PhysicalDomain=network_engine_domain  SubClassName=ps_output  LeftPortType=input  RightPortType=output  PseudoPeriodic=off  Frequencies=[]  VectorFormat=1-D array  Unit=degC  AffineConversion=on
  Temperature Sensor : fl_lib/Thermal/Thermal Sensors/Temperature Sensor  temperature_measure=foundation.enum.MeasurementReference.difference
  ThRef : fl_lib/Thermal/Thermal Elements/Thermal Reference
  H : PMIOPort  Side=Left
  tag scope: TR_eq=global
  wires:
  PS-Simulink Converter/1 -> [TR_eq]
  connections:
  Temperature Sensor/RConn2 -- PS-Simulink Converter/LConn1
  ThRef/LConn1 -- Temperature Sensor/RConn1
  H/RConn1 -- Temperature Sensor/LConn1

== system PMSM_temperature_estimation_EKF/Equivalent Model/Sensing Temperature WiA ==
  PS-Simulink Converter : nesl_utility/PS-Simulink Converter  PhysicalDomain=network_engine_domain  SubClassName=ps_output  LeftPortType=input  RightPortType=output  PseudoPeriodic=off  Frequencies=[]  VectorFormat=1-D array  Unit=degC  AffineConversion=on
  Temperature Sensor : fl_lib/Thermal/Thermal Sensors/Temperature Sensor  temperature_measure=foundation.enum.MeasurementReference.difference
  ThRef : fl_lib/Thermal/Thermal Elements/Thermal Reference
  H : PMIOPort  Side=Left
  tag scope: TA_eq=global
  wires:
  PS-Simulink Converter/1 -> [TA_eq]
  connections:
  H/RConn1 -- Temperature Sensor/LConn1
  Temperature Sensor/RConn2 -- PS-Simulink Converter/LConn1
  Temperature Sensor/RConn1 -- ThRef/LConn1

== system PMSM_temperature_estimation_EKF/Equivalent Model/Sensing Temperature WiB ==
  PS-Simulink Converter : nesl_utility/PS-Simulink Converter  PhysicalDomain=network_engine_domain  SubClassName=ps_output  LeftPortType=input  RightPortType=output  PseudoPeriodic=off  Frequencies=[]  VectorFormat=1-D array  Unit=degC  AffineConversion=on
  Temperature Sensor : fl_lib/Thermal/Thermal Sensors/Temperature Sensor  temperature_measure=foundation.enum.MeasurementReference.difference
  ThRef2 : fl_lib/Thermal/Thermal Elements/Thermal Reference
  H : PMIOPort  Side=Left
  tag scope: TB_eq=global
  wires:
  PS-Simulink Converter/1 -> [TB_eq]
  connections:
  Temperature Sensor/RConn2 -- PS-Simulink Converter/LConn1
  H/RConn1 -- Temperature Sensor/LConn1
  Temperature Sensor/RConn1 -- ThRef2/LConn1

== system PMSM_temperature_estimation_EKF/Equivalent Model/Sensing Temperature WiC ==
  PS-Simulink Converter : nesl_utility/PS-Simulink Converter  PhysicalDomain=network_engine_domain  SubClassName=ps_output  LeftPortType=input  RightPortType=output  PseudoPeriodic=off  Frequencies=[]  VectorFormat=1-D array  Unit=degC  AffineConversion=on
  Temperature Sensor : fl_lib/Thermal/Thermal Sensors/Temperature Sensor  temperature_measure=foundation.enum.MeasurementReference.difference
  ThRef : fl_lib/Thermal/Thermal Elements/Thermal Reference
  H : PMIOPort  Side=Left
  tag scope: TC_eq=global
  wires:
  PS-Simulink Converter/1 -> [TC_eq]
  connections:
  H/RConn1 -- Temperature Sensor/LConn1
  ThRef/LConn1 -- Temperature Sensor/RConn1
  Temperature Sensor/RConn2 -- PS-Simulink Converter/LConn1

== system PMSM_temperature_estimation_EKF/Low-freq Model/Sensing Temperature Rot ==
  PS-Simulink Converter : nesl_utility/PS-Simulink Converter  PhysicalDomain=network_engine_domain  SubClassName=ps_output  LeftPortType=input  RightPortType=output  PseudoPeriodic=off  Frequencies=[]  VectorFormat=1-D array  Unit=degC  AffineConversion=on
  Temperature Sensor : fl_lib/Thermal/Thermal Sensors/Temperature Sensor  temperature_measure=foundation.enum.MeasurementReference.difference
  ThRef : fl_lib/Thermal/Thermal Elements/Thermal Reference
  H : PMIOPort  Side=Left
  tag scope: TR_lf=global
  wires:
  PS-Simulink Converter/1 -> [TR_lf]
  connections:
  Temperature Sensor/RConn2 -- PS-Simulink Converter/LConn1
  ThRef/LConn1 -- Temperature Sensor/RConn1
  H/RConn1 -- Temperature Sensor/LConn1

== system PMSM_temperature_estimation_EKF/Low-freq Model/Sensing Temperature WiA ==
  PS-Simulink Converter : nesl_utility/PS-Simulink Converter  PhysicalDomain=network_engine_domain  SubClassName=ps_output  LeftPortType=input  RightPortType=output  PseudoPeriodic=off  Frequencies=[]  VectorFormat=1-D array  Unit=degC  AffineConversion=on
  Temperature Sensor : fl_lib/Thermal/Thermal Sensors/Temperature Sensor  temperature_measure=foundation.enum.MeasurementReference.difference
  ThRef : fl_lib/Thermal/Thermal Elements/Thermal Reference
  H : PMIOPort  Side=Left
  tag scope: TA_lf=global
  wires:
  PS-Simulink Converter/1 -> [TA_lf]
  connections:
  H/RConn1 -- Temperature Sensor/LConn1
  Temperature Sensor/RConn2 -- PS-Simulink Converter/LConn1
  Temperature Sensor/RConn1 -- ThRef/LConn1

== system PMSM_temperature_estimation_EKF/Low-freq Model/Sensing Temperature WiB ==
  PS-Simulink Converter : nesl_utility/PS-Simulink Converter  PhysicalDomain=network_engine_domain  SubClassName=ps_output  LeftPortType=input  RightPortType=output  PseudoPeriodic=off  Frequencies=[]  VectorFormat=1-D array  Unit=degC  AffineConversion=on
  Temperature Sensor : fl_lib/Thermal/Thermal Sensors/Temperature Sensor  temperature_measure=foundation.enum.MeasurementReference.difference
  ThRef2 : fl_lib/Thermal/Thermal Elements/Thermal Reference
  H : PMIOPort  Side=Left
  tag scope: TB_lf=global
  wires:
  PS-Simulink Converter/1 -> [TB_lf]
  connections:
  Temperature Sensor/RConn2 -- PS-Simulink Converter/LConn1
  H/RConn1 -- Temperature Sensor/LConn1
  Temperature Sensor/RConn1 -- ThRef2/LConn1

== system PMSM_temperature_estimation_EKF/Low-freq Model/Sensing Temperature WiC ==
  PS-Simulink Converter : nesl_utility/PS-Simulink Converter  PhysicalDomain=network_engine_domain  SubClassName=ps_output  LeftPortType=input  RightPortType=output  PseudoPeriodic=off  Frequencies=[]  VectorFormat=1-D array  Unit=degC  AffineConversion=on
  Temperature Sensor : fl_lib/Thermal/Thermal Sensors/Temperature Sensor  temperature_measure=foundation.enum.MeasurementReference.difference
  ThRef : fl_lib/Thermal/Thermal Elements/Thermal Reference
  H : PMIOPort  Side=Left
  tag scope: TC_lf=global
  wires:
  PS-Simulink Converter/1 -> [TC_lf]
  connections:
  H/RConn1 -- Temperature Sensor/LConn1
  ThRef/LConn1 -- Temperature Sensor/RConn1
  Temperature Sensor/RConn2 -- PS-Simulink Converter/LConn1

== system PMSM_temperature_estimation_EKF/Low-freq Simplified Model/Sensing Temperature Rotor ==
  PS-Simulink Converter : nesl_utility/PS-Simulink Converter  PhysicalDomain=network_engine_domain  SubClassName=ps_output  LeftPortType=input  RightPortType=output  PseudoPeriodic=off  Frequencies=[]  VectorFormat=1-D array  Unit=degC  AffineConversion=on
  Temperature Sensor : fl_lib/Thermal/Thermal Sensors/Temperature Sensor  temperature_measure=foundation.enum.MeasurementReference.difference
  ThRef : fl_lib/Thermal/Thermal Elements/Thermal Reference
  H : PMIOPort  Side=Left
  tag scope: TR_lfs=global
  wires:
  PS-Simulink Converter/1 -> [TR_lfs]
  connections:
  Temperature Sensor/RConn2 -- PS-Simulink Converter/LConn1
  ThRef/LConn1 -- Temperature Sensor/RConn1
  H/RConn1 -- Temperature Sensor/LConn1

== system PMSM_temperature_estimation_EKF/Low-freq Simplified Model/Sensing Temperature Wire ==
  PS-Simulink Converter : nesl_utility/PS-Simulink Converter  PhysicalDomain=network_engine_domain  SubClassName=ps_output  LeftPortType=input  RightPortType=output  PseudoPeriodic=off  Frequencies=[]  VectorFormat=1-D array  Unit=degC  AffineConversion=on
  Temperature Sensor : fl_lib/Thermal/Thermal Sensors/Temperature Sensor  temperature_measure=foundation.enum.MeasurementReference.difference
  ThRef2 : fl_lib/Thermal/Thermal Elements/Thermal Reference
  H : PMIOPort  Side=Left
  tag scope: TW_lfs=global
  wires:
  PS-Simulink Converter/1 -> [TW_lfs]
  connections:
  Temperature Sensor/RConn2 -- PS-Simulink Converter/LConn1
  H/RConn1 -- Temperature Sensor/LConn1
  Temperature Sensor/RConn1 -- ThRef2/LConn1

== system PMSM_temperature_estimation_EKF/PMSM Controller/Vector controller ==
  trqRef : Inport
  theta : Inport  Port=2
  I_abc : Inport  Port=3
  Convert from mechanical to electrical angle : Gain  Gain=Np  SaturateOnIntegerOverflow=on  OutDataTypeStr=Inherit: Same as input  ParamDataTypeStr=Inherit: Same as input
  Current control and gate assignment (averaged) : Subsystem  VariantControl=Variant1
  Inverse Park's : Subsystem
  Map torque demand to equivalent Iq value : Gain  Gain=2/(3*Np*lambda)  SaturateOnIntegerOverflow=on  OutDataTypeStr=Inherit: Same as input  ParamDataTypeStr=Inherit: Same as input
  G : Outport  VectorParamsAs1DForOutWhenUnconnected=off
  wires:
  Current control and gate assignment (averaged)/1(G) -> G/1
  I_abc/1 -> Current control and gate assignment (averaged)/2(iABC)
  trqRef/1 -> Map torque demand to equivalent Iq value/1
  Map torque demand to equivalent Iq value/1 -> Inverse Park's/1(iqRef)
  theta/1 -> Convert from mechanical to electrical angle/1
  Convert from mechanical to electrical angle/1 -> Inverse Park's/2(theta)
  Inverse Park's/1(iRef) -> Current control and gate assignment (averaged)/1(iRefABC)

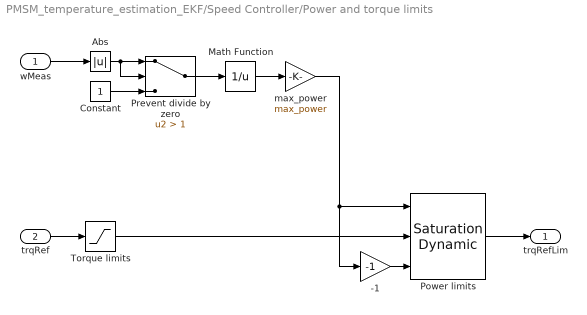
== system PMSM_temperature_estimation_EKF/Speed Controller/Power and torque limits ==
  wMeas : Inport
  trqRef : Inport  Port=2
  -1 : Gain  Gain=-1
  Abs : Abs  SaturateOnIntegerOverflow=off
  Constant : Constant  SampleTime=dt_speed_control
  Math Function : Math  Operator=reciprocal  SignedPower=on
  Power limits : simulink/Discontinuities/Saturation Dynamic  OutMin=[]  OutMax=[]  OutDataTypeStr=Inherit: Same as second input  OutDataType=fixdt(1, 16)  OutScaling=2^-10  DoSatur=off
  Prevent divide by zero : Switch  Criteria=u2 > Threshold  Threshold=1  SaturateOnIntegerOverflow=off  InputSameDT=off
  Torque limits : Saturate  UpperLimit=max_torque  LowerLimit=-max_torque
  max_power : Gain  Gain=max_power
  trqRefLim : Outport  VectorParamsAs1DForOutWhenUnconnected=off
  wires:
  wMeas/1 -> Abs/1
  -1/1 -> Power limits/3
  Constant/1 -> Prevent divide by zero/3
  Prevent divide by zero/1 -> Math Function/1
  max_power/1 -> -1/1, Power limits/1
  Math Function/1 -> max_power/1
  Torque limits/1 -> Power limits/2
  Abs/1 -> Prevent divide by zero/1, Prevent divide by zero/2
  trqRef/1 -> Torque limits/1
  Power limits/1 -> trqRefLim/1

== system PMSM_temperature_estimation_EKF/Speed Controller/Speed controller ==
  wMeas : Inport
  wRef : Inport  Port=2
  Speed controller : Subsystem  mask(P+I motor speed controller){Kp=300, Ki=300, trqMax=max_torque, ts=dt_speed_control}
      mask prompts: Kp "Proportional gain (Nm/(rad/s))"; Ki "Integral gain (Nm/rad)"; trqMax "Maximum torque demand"; ts "Sample time"
      mask help: Inputs wRef and wMeas are the demanded rotor speed and measured rotor speed in rad/s. The controller output is a torque demand in Nm.
  trqRef : Outport  VectorParamsAs1DForOutWhenUnconnected=off
  tag scope: wDemand=global
  wires:
  wRef/1 -> Speed controller/1(wRef), [wDemand]
  Speed controller/1(trqRef) -> trqRef/1
  wMeas/1 -> Speed controller/2(wMeas)
